simulink model "Problem_52S"  (R2018b)
settings: Solver=VariableStepAuto  StartTime=0.0  StopTime=20  RelTol=1e-3
values from neighbouring files (symbols this model uses):
  poly_block_52M = [-27/800, 27/80, 0,0]    [hw7_main.m]
libraries: cstblocks x1
settings Model: Creator=HyperDrive  LastModifiedBy=HyperDrive

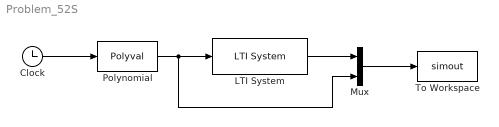
== system Problem_52S ==
  Clock : Clock
  LTI System : cstblocks/LTI System  sys=LTI_52M  IC=[]
  Mux : Mux  Inputs=2
  Polynomial : Polyval  Coefs=poly_block_52M
  To Workspace : ToWorkspace  VariableName=simout  SaveFormat=Timeseries  SampleTime=-1
  wires:
  Clock/1 -> Polynomial/1
  Polynomial/1 -> Mux/2, LTI System/1
  LTI System/1 -> Mux/1
  Mux/1 -> To Workspace/1
